simulink model "sim_2_5"  (R2023b)
settings: Solver=FixedStepAuto  StartTime=0.0  StopTime=50  FixedStep=Ts  RelTol=1e-3
values from neighbouring files (symbols this model uses):
  k1 = 1    [H2_5.m]
  k2 = 1    [H2_5.m]
  k3 = 0.2    [H2_5.m]
  qi = [1 1 pi/4]    [H2_5.m]
  Ts = 0.05    [H2_5.m]
libraries: robotmobilelib x1
settings Model: Creator=Valentina Giannotti  LastModifiedBy=Valentina Giannotti

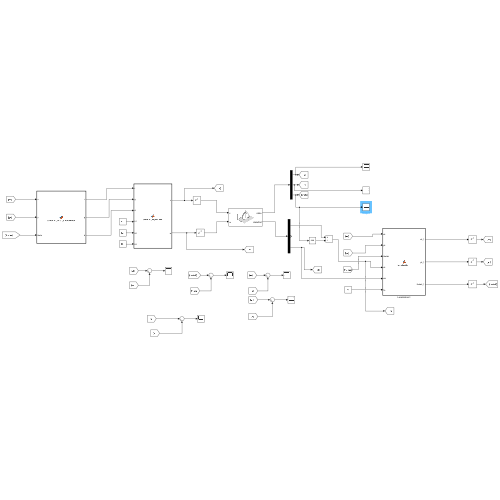
[thumbnail: Simulink's stored preview of the top-level diagram]
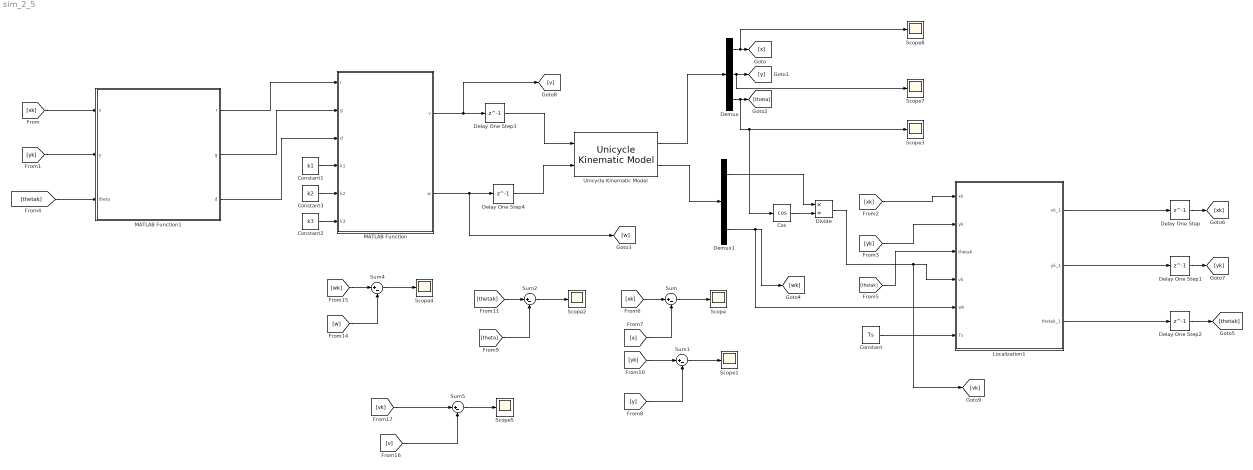
== system sim_2_5 ==
  Constant : Constant  Value=Ts
  Constant1 : Constant  Value=k1
  Constant2 : Constant  Value=k3
  Constant3 : Constant  Value=k2
  Cos : Trigonometry  Operator=cos
  Delay One Step : Delay  DelayLength=1  InitialCondition=qi(1)
  Delay One Step1 : Delay  DelayLength=1  InitialCondition=qi(2)
  Delay One Step2 : Delay  DelayLength=1  InitialCondition=qi(3)
  Delay One Step3 : Delay  DelayLength=1  InitialCondition=0
  Delay One Step4 : Delay  DelayLength=1  InitialCondition=0
  Demux : Demux  Outputs=3
  Demux1 : Demux  Outputs=3
  Divide : Product  Inputs=*/
  Localization1 : MATLAB Function  TreatAsAtomicUnit=on
  MATLAB Function : MATLAB Function  TreatAsAtomicUnit=on
  MATLAB Function1 : MATLAB Function  TreatAsAtomicUnit=on
  Scope{,1..5,7..8} (8 alike) : Scope
  Sum{,1..2,4..5} (5 alike) : Sum  Inputs=|+-
  Unicycle Kinematic Model : robotmobilelib/Unicycle Kinematic Model  VehicleInputs=Vehicle Speed & Heading Angular Velocity  WheelRadius=0.1  WheelSpeedRange=[-Inf Inf]  InitialState=qi  SimulateUsing=Interpreted execution
  wires:
  Demux/3 -> Cos/1, Scope3/1, [theta]
  Demux/2 -> Scope7/1, [y]
  Demux/1 -> Scope8/1, [x]
  Unicycle Kinematic Model/1 -> Demux/1
  [xk] -> MATLAB Function1/1(x)
  [yk] -> MATLAB Function1/2(y)
  [thetak] -> MATLAB Function1/3(theta)
  MATLAB Function1/1(r) -> MATLAB Function/1(r)
  MATLAB Function1/3(d) -> MATLAB Function/3(d)
  MATLAB Function1/2(g) -> MATLAB Function/2(g)
  Delay One Step2/1 -> [thetak]
  Delay One Step1/1 -> [yk]
  Delay One Step/1 -> [xk]
  Localization1/1(xk_1) -> Delay One Step/1
  Localization1/2(yk_1) -> Delay One Step1/1
  Localization1/3(thetak_1) -> Delay One Step2/1
  [xk] -> Localization1/1(xk)
  [yk] -> Localization1/2(yk)
  [thetak] -> Localization1/3(thetak)
  Demux1/3 -> Localization1/5(wk), [wk]
  Constant/1 -> Localization1/6(Ts)
  Cos/1 -> Divide/2
  Constant1/1 -> MATLAB Function/4(k1)
  Constant3/1 -> MATLAB Function/5(k2)
  Constant2/1 -> MATLAB Function/6(k3)
  [xk] -> Sum/1
  [x] -> Sum/2
  Sum/1 -> Scope/1
  Sum1/1 -> Scope1/1
  [y] -> Sum1/2
  [yk] -> Sum1/1
  Sum2/1 -> Scope2/1
  [theta] -> Sum2/2
  [thetak] -> Sum2/1
  Demux1/1 -> Divide/1
  MATLAB Function/1(v) -> Delay One Step3/1, [v]
  Delay One Step3/1 -> Unicycle Kinematic Model/1
  MATLAB Function/2(w) -> Delay One Step4/1, [w]
  Delay One Step4/1 -> Unicycle Kinematic Model/2
  Sum4/1 -> Scope4/1
  [w] -> Sum4/2
  [wk] -> Sum4/1
  [v] -> Sum5/2
  [vk] -> Sum5/1
  Sum5/1 -> Scope5/1
  Unicycle Kinematic Model/2 -> Demux1/1
  Divide/1 -> [vk], Localization1/4(vk)

== matlab function sim_2_5/MATLAB Function1 ==
  data: x input; r output; g output; y input; theta input; d output
function [r,g,d] = compute_polar_coordinates(x,y,theta)

r=sqrt(x^2+y^2);
g=atan2(y,x)-theta+pi;
d=g+theta;

end

== matlab function sim_2_5/MATLAB Function ==
  data: r input; v output; w output; g input; d input; k1 input; k2 input; k3 input
function [v,w] = posture_regulation(r,g,d, k1, k2, k3)


v=k1*r*cos(g);
w=k2*g+k1*sin(g)*cos(g)*(1+k3*d/g);

end

== matlab function sim_2_5/Localization1 ==
  data: xk input; yk input; thetak input; xk_1 output; yk_1 output; thetak_1 output; vk input; wk input; Ts input
function [xk_1,yk_1,thetak_1] = Localization1(xk, yk, thetak, vk, wk, Ts)

xk_1=xk+vk*Ts*cos(thetak+wk*Ts/2);
yk_1=yk+vk*Ts*sin(thetak+wk*Ts/2);
thetak_1=thetak+wk*Ts;

end
